simulink model "scdtopmdl"  (Simulink 7.6)
settings: Solver=ode45  StartTime=0.0  StopTime=10.0  RelTol=1e-3
settings Model: Creator=The MathWorks Inc.
settings DebuggingCC: SolverPrmCheckMsg=none  StrictBusMsg=Warning

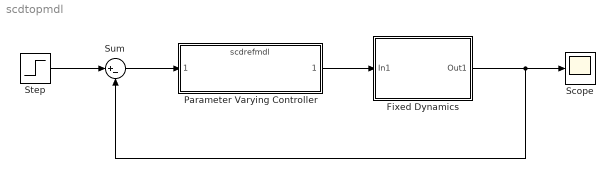
== system scdtopmdl ==
  Fixed Dynamics : Subsystem
  Parameter Varying Controller : ModelReference  ModelNameDialog=scdrefmdl  SimulationMode=Normal  ModelReferenceVersion=1.9  CopyOfModelName=scdrefmdl
  Scope : Scope
  Step : Step  SampleTime=0
  Sum : Sum  Inputs=|+-
  wires:
  Step/1 -> Sum/1
  Sum/1 -> Parameter Varying Controller/1
  Parameter Varying Controller/1 -> Fixed Dynamics/1(In1)
  Fixed Dynamics/1(Out1) -> Sum/2, Scope/1

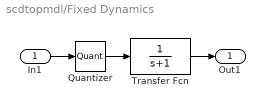
== system scdtopmdl/Fixed Dynamics ==
  In1 : Inport
  Quantizer : Quantizer
  Transfer Fcn : TransferFcn  Denominator=[1 1]
  Out1 : Outport
  wires:
  In1/1 -> Quantizer/1
  Transfer Fcn/1 -> Out1/1
  Quantizer/1 -> Transfer Fcn/1
